simulink model "LKAS_AutoSave_DF_20220414_1924_SW62"  (R2018b)
settings: Solver=FixedStepDiscrete  StartTime=0.0  StopTime=10.0  FixedStep=0.01  RelTol=1e-3
model workspace (MAT data in the model file):
  MCOS : class17 (value not decoded)
  MCOS : class17 (value not decoded)
  MCOS : class17 (value not decoded)
  MCOS : class17 (value not decoded)
  MCOS : class17 (value not decoded)
  MCOS : class17 (value not decoded)
  MCOS : class17 (value not decoded)
  MCOS : class17 (value not decoded)
  MCOS : class17 (value not decoded)
  MCOS : class17 (value not decoded)
  MCOS : class17 (value not decoded)
  MCOS : class17 (value not decoded)
  MCOS : class17 (value not decoded)
  MCOS : class17 (value not decoded)
  MCOS : class17 (value not decoded)
  MCOS : class17 (value not decoded)
  MCOS : class17 (value not decoded)
  MCOS : class17 (value not decoded)
  MCOS : class17 (value not decoded)
  MCOS : class17 (value not decoded)
  MCOS : class17 (value not decoded)
  MCOS : class17 (value not decoded)
  MCOS : class17 (value not decoded)
  MCOS : class17 (value not decoded)
  MCOS : class17 (value not decoded)
  MCOS : class17 (value not decoded)
  MCOS : class17 (value not decoded)
  MCOS : class17 (value not decoded)
  MCOS : class17 (value not decoded)
  MCOS : class17 (value not decoded)
  MCOS : class17 (value not decoded)
  MCOS : class17 (value not decoded)
  MCOS : class17 (value not decoded)
  MCOS : class17 (value not decoded)
  MCOS : class17 (value not decoded)
  MCOS : class17 (value not decoded)
  MCOS : class17 (value not decoded)
  MCOS : class17 (value not decoded)
  MCOS : class17 (value not decoded)
  MCOS : class17 (value not decoded)
  MCOS : class17 (value not decoded)
  MCOS : class17 (value not decoded)
  MCOS : class17 (value not decoded)
  MCOS : class17 (value not decoded)
  MCOS : class17 (value not decoded)
  MCOS : class17 (value not decoded)
  MCOS : class17 (value not decoded)
  MCOS : class17 (value not decoded)
  MCOS : class17 (value not decoded)
  MCOS : class17 (value not decoded)
  MCOS : class17 (value not decoded)
  MCOS : class17 (value not decoded)
  MCOS : class17 (value not decoded)
  MCOS : class17 (value not decoded)
  MCOS : class17 (value not decoded)
  MCOS : class17 (value not decoded)
  MCOS : class17 (value not decoded)
  MCOS : class17 (value not decoded)
  MCOS : class17 (value not decoded)
  MCOS : class17 (value not decoded)
  MCOS : class17 (value not decoded)
  MCOS : class17 (value not decoded)
  MCOS : class17 (value not decoded)
  MCOS : class17 (value not decoded)
  MCOS : class17 (value not decoded)
  MCOS : class17 (value not decoded)
  MCOS : class17 (value not decoded)
  MCOS : class17 (value not decoded)
  MCOS : class17 (value not decoded)
  MCOS : class17 (value not decoded)
  MCOS : class17 (value not decoded)
  MCOS : class17 (value not decoded)
  MCOS : class17 (value not decoded)
  MCOS : class17 (value not decoded)
  MCOS : class17 (value not decoded)
  MCOS : class17 (value not decoded)
  MCOS : class17 (value not decoded)
  MCOS : class17 (value not decoded)
  MCOS : class17 (value not decoded)
  MCOS : class17 (value not decoded)
  MCOS : class17 (value not decoded)
  MCOS : class17 (value not decoded)
  MCOS : class17 (value not decoded)
  MCOS : class17 (value not decoded)
  MCOS : class17 (value not decoded)
  MCOS : class17 (value not decoded)
  MCOS : class17 (value not decoded)
  MCOS : class17 (value not decoded)
  MCOS : class17 (value not decoded)
  MCOS : class17 (value not decoded)
  MCOS : class17 (value not decoded)
  MCOS : class17 (value not decoded)
  MCOS : class17 (value not decoded)
  MCOS : class17 (value not decoded)
  MCOS : class17 (value not decoded)
  MCOS : class17 (value not decoded)
  MCOS : class17 (value not decoded)
  MCOS : class17 (value not decoded)
  MCOS : class17 (value not decoded)
  MCOS : class17 (value not decoded)
  MCOS : class17 (value not decoded)
  MCOS : class17 (value not decoded)
  MCOS : class17 (value not decoded)
  MCOS : class17 (value not decoded)
  MCOS : class17 (value not decoded)
  MCOS : class17 (value not decoded)
  MCOS : class17 (value not decoded)
  MCOS : class17 (value not decoded)
  MCOS : class17 (value not decoded)
undefined symbols (not defined in the file): LKA_CarWidth, LKA_SampleTime, LKA_StrRatio_C, LKA_Veh2CamL_C, LKA_Veh2CamW_C, LKA_WhlBaseL_C, LL_CompHdAg_C, LL_CompSWA_C, LL_CrvtPrvwT_C, LL_DesDvt_C, LL_DvtComp_C, LL_DvtPrvwT_C, LL_DvtSpdDet_vDvtSpdMin_C, LL_HandsOff_ExitTime, LL_HandsOff_TextTime, LL_HandsOff_WarnTime, LL_HdAgExT_C, LL_HdAgPrvwT_C, LL_LAccMax_C, LL_LAccRMax_C, LL_LDW_EarliestWarnLine_C, LL_LDW_LatestWarnLine_C, LL_LDWS_SUPPRESS_HEADING, LL_LFClb_TFC_FfCtlRatio_C, LL_LFClb_TFC_KdBalance_C, LL_LFClb_TFC_KdMaxSWA_C, LL_LFClb_TFC_KdV1_C, LL_LFClb_TFC_KdV2_C, LL_LFClb_TFC_KdVehSpdLwr_C, LL_LFClb_TFC_KdVehSpdUpr_C, LL_LFClb_TFC_Ki_C, LL_LFClb_TFC_KiMaxSWA_C, LL_LFClb_TFC_Kp_C, LL_LFClb_TFC_KpKlat_C, LL_LFClb_TFC_KpV1_C, LL_LFClb_TFC_KpV2_C, LL_LFClb_TFC_KpVehSpdLwr_C, LL_LFClb_TFC_KpVehSpdUpr_C, LL_LFClb_TFC_PrvwT_C, LL_LKA_EarliestWarnLine_C, LL_LKA_EnableLine_DvtMax, LL_LKA_EnableLine_DvtMin, LL_LKA_EnableLine_Max, LL_LKA_LatestWarnLine_C, LL_LKAExPrcs_ExitC0Dvt, LL_LKAExPrcs_ExitC0Swt, LL_LKAExPrcs_tiExitDelayTime3, LL_LKAExPrcs_tiExitTime1, LL_LKAExPrcs_tiExitTime2, LL_LKAExPrcs_tiExitTime3, LL_LKAS_OUT_OF_CONTROL_LAT_VEL, LL_LKAS_OUT_OF_CONTROL_TTLC, LL_LKASWASyn_M0, LL_LKASWASyn_M1, LL_LKASWASyn_M2, LL_LKASWASyn_M3D, LL_LKASWASyn_M3K_DT, LL_LKASWASyn_M3K_MSD, LL_LKASWASyn_M4K, LL_LKASWASyn_SWAaddMax ... (+50)
libraries: simulink x234, canmsglib x6, dspstat3 x3, simulink_extras x1
(part 12 of 17)

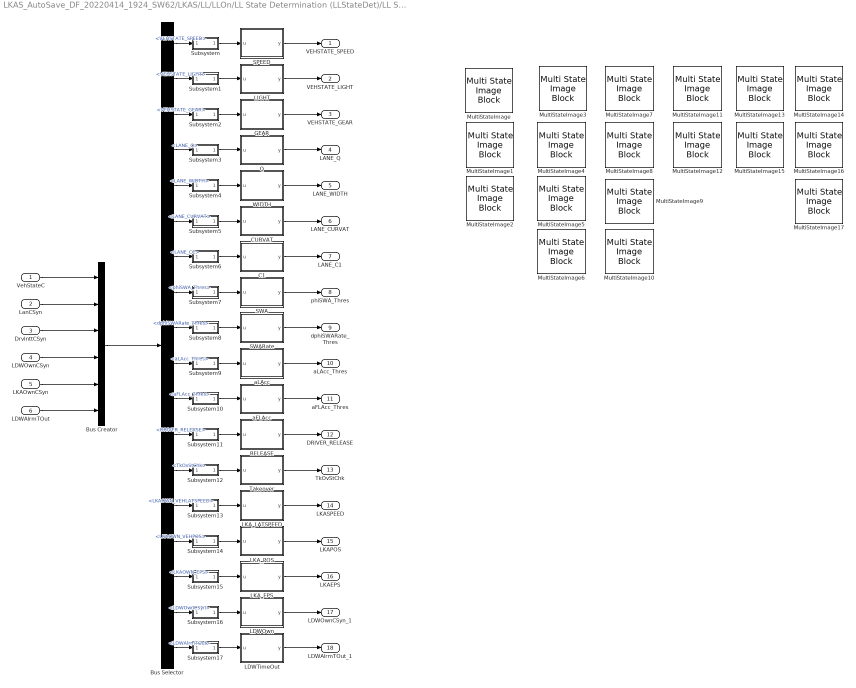
== system LKAS_AutoSave_DF_20220414_1924_SW62/LKAS/LL/LLOn/LL State Determination (LLStateDet)/LL State Machine Conditions (LLSMCon)/Disable Condition (DisblC)/Subsystem ==
  VehStateC : Inport
  LanCSyn : Inport  Port=2
  DrvInttCSyn : Inport  Port=3
  LDWOwnCSyn : Inport  Port=4
  LKAOwnCSyn : Inport  Port=5
  LDWAlrmTOut : Inport  Port=6
  Bus Creator : BusCreator  Inputs=6
  Bus Selector : BusSelector  OutputSignals=VehStateC.VEHSTATE_SPEED,VehStateC.VEHSTATE_LIGHT,VehStateC.VEHSTATE_GEAR,LaneCSyn.LANE_Q,LaneCSyn.LANE_WIDTH,LaneCSyn.LANE_CURVAT,LaneCSyn.LANE_C1,DrvInttCSyn.DrvActnDet.phiSWA_Thres,DrvInttCSyn.DrvActnDet.dphiSWARate_Thres,DrvInttCSyn.DrvActnDet.aLAcc_Thres,DrvInttCSyn.DrvActnDet.aFLAcc_Thres,DrvInttCSyn.DRIVER_RELEASE,DrvInttCSyn.TkOvStChk,LKAOwnSyn.LKAOWN_VEHLATSPEED,LKAOwnSyn.LKAOWN_VEHPOS,LKAOwnSyn.LKAOWN_EPS,LDWOwnCSyn,LDWAlrmTOut
  C1 : MATLAB Function  TreatAsAtomicUnit=on
  CURVAT : MATLAB Function  TreatAsAtomicUnit=on
  GEAR : MATLAB Function  TreatAsAtomicUnit=on
  LDWOwn : MATLAB Function  TreatAsAtomicUnit=on
  LDWTimeOut : MATLAB Function  TreatAsAtomicUnit=on
  LIGHT : MATLAB Function  TreatAsAtomicUnit=on
  LKA_EPS : MATLAB Function  TreatAsAtomicUnit=on
  LKA_LATSPEED : MATLAB Function  TreatAsAtomicUnit=on
  LKA_POS : MATLAB Function  TreatAsAtomicUnit=on
  MultiStateImage : MultiStateImageBlock  WebBlockId=3772
  MultiStateImage1 : MultiStateImageBlock  WebBlockId=3773
  MultiStateImage10 : MultiStateImageBlock  WebBlockId=3774
  MultiStateImage11 : MultiStateImageBlock  WebBlockId=3775
  MultiStateImage12 : MultiStateImageBlock  WebBlockId=3776
  MultiStateImage13 : MultiStateImageBlock  WebBlockId=3777
  MultiStateImage14 : MultiStateImageBlock  WebBlockId=3778
  MultiStateImage15 : MultiStateImageBlock  WebBlockId=3779
  MultiStateImage16 : MultiStateImageBlock  WebBlockId=3780
  MultiStateImage17 : MultiStateImageBlock  WebBlockId=3781
  MultiStateImage2 : MultiStateImageBlock  WebBlockId=3782
  MultiStateImage3 : MultiStateImageBlock  WebBlockId=3783
  MultiStateImage4 : MultiStateImageBlock  WebBlockId=3784
  MultiStateImage5 : MultiStateImageBlock  WebBlockId=3785
  MultiStateImage6 : MultiStateImageBlock  WebBlockId=3786
  MultiStateImage7 : MultiStateImageBlock  WebBlockId=3787
  MultiStateImage8 : MultiStateImageBlock  WebBlockId=3788
  MultiStateImage9 : MultiStateImageBlock  WebBlockId=3789
  Q : MATLAB Function  TreatAsAtomicUnit=on
  RELEASE : MATLAB Function  TreatAsAtomicUnit=on
  SPEED : MATLAB Function  TreatAsAtomicUnit=on
  SWA : MATLAB Function  TreatAsAtomicUnit=on
  SWARate : MATLAB Function  TreatAsAtomicUnit=on
  Subsystem : Subsystem
  Subsystem1 : Subsystem
  Subsystem10 : Subsystem
  Subsystem11 : Subsystem
  Subsystem12 : Subsystem
  Subsystem13 : Subsystem
  Subsystem14 : Subsystem
  Subsystem15 : Subsystem
  Subsystem16 : Subsystem
  Subsystem17 : Subsystem
  Subsystem2 : Subsystem
  Subsystem3 : Subsystem
  Subsystem4 : Subsystem
  Subsystem5 : Subsystem
  Subsystem6 : Subsystem
  Subsystem7 : Subsystem
  Subsystem8 : Subsystem
  Subsystem9 : Subsystem
  Takeover : MATLAB Function  TreatAsAtomicUnit=on
  WIDTH : MATLAB Function  TreatAsAtomicUnit=on
  aFLAcc : MATLAB Function  TreatAsAtomicUnit=on
  aLAcc : MATLAB Function  TreatAsAtomicUnit=on
  VEHSTATE_SPEED : Outport
  VEHSTATE_LIGHT : Outport  Port=2
  VEHSTATE_GEAR : Outport  Port=3
  LANE_Q : Outport  Port=4
  LANE_WIDTH : Outport  Port=5
  LANE_CURVAT : Outport  Port=6
  LANE_C1 : Outport  Port=7
  phiSWA_Thres : Outport  Port=8
  dphiSWARate_Thres : Outport  Port=9
  aLAcc_Thres : Outport  Port=10
  aFLAcc_Thres : Outport  Port=11
  DRIVER_RELEASE : Outport  Port=12
  TkOvStChk : Outport  Port=13
  LKASPEED : Outport  Port=14
  LKAPOS : Outport  Port=15
  LKAEPS : Outport  Port=16
  LDWOwnCSyn_1 : Outport  Port=17
  LDWAlrmTOut_1 : Outport  Port=18
  wires:
  Bus Selector/16 -> Subsystem15/1(in1)  "<LKAOWN_EPS>"
  Subsystem15/1(Out1) -> LKA_EPS/1(u)
  LKA_EPS/1(y) -> LKAEPS/1
  Bus Selector/14 -> Subsystem13/1(in1)  "<LKAOWN_VEHLATSPEED>"
  Subsystem13/1(Out1) -> LKA_LATSPEED/1(u)
  LKA_LATSPEED/1(y) -> LKASPEED/1
  Subsystem17/1(Out1) -> LDWTimeOut/1(u)
  Subsystem14/1(Out1) -> LKA_POS/1(u)
  Subsystem16/1(Out1) -> LDWOwn/1(u)
  Subsystem11/1(Out1) -> RELEASE/1(u)
  Subsystem12/1(Out1) -> Takeover/1(u)
  Subsystem10/1(Out1) -> aFLAcc/1(u)
  Subsystem9/1(Out1) -> aLAcc/1(u)
  Subsystem8/1(Out1) -> SWARate/1(u)
  Subsystem7/1(Out1) -> SWA/1(u)
  Subsystem6/1(Out1) -> C1/1(u)
  Subsystem5/1(Out1) -> CURVAT/1(u)
  Subsystem4/1(Out1) -> WIDTH/1(u)
  Subsystem3/1(Out1) -> Q/1(u)
  Subsystem2/1(Out1) -> GEAR/1(u)
  Subsystem1/1(Out1) -> LIGHT/1(u)
  Subsystem/1(Out1) -> SPEED/1(u)
  Bus Selector/1 -> Subsystem/1(in1)  "<VEHSTATE_SPEED>"
  SPEED/1(y) -> VEHSTATE_SPEED/1
  LIGHT/1(y) -> VEHSTATE_LIGHT/1
  GEAR/1(y) -> VEHSTATE_GEAR/1
  aLAcc/1(y) -> aLAcc_Thres/1
  WIDTH/1(y) -> LANE_WIDTH/1
  LDWTimeOut/1(y) -> LDWAlrmTOut_1/1
  SWA/1(y) -> phiSWA_Thres/1
  aFLAcc/1(y) -> aFLAcc_Thres/1
  LDWAlrmTOut/1 -> Bus Creator/6
  Bus Selector/6 -> Subsystem5/1(in1)  "<LANE_CURVAT>"
  RELEASE/1(y) -> DRIVER_RELEASE/1
  SWARate/1(y) -> dphiSWARate_Thres/1
  Bus Selector/3 -> Subsystem2/1(in1)  "<VEHSTATE_GEAR>"
  LDWOwnCSyn/1 -> Bus Creator/4
  DrvInttCSyn/1 -> Bus Creator/3
  Bus Selector/5 -> Subsystem4/1(in1)  "<LANE_WIDTH>"
  C1/1(y) -> LANE_C1/1
  LanCSyn/1 -> Bus Creator/2
  Takeover/1(y) -> TkOvStChk/1
  Bus Selector/7 -> Subsystem6/1(in1)  "<LANE_C1>"
  Bus Selector/9 -> Subsystem8/1(in1)  "<dphiSWARate_Thres>"
  Bus Selector/2 -> Subsystem1/1(in1)  "<VEHSTATE_LIGHT>"
  Q/1(y) -> LANE_Q/1
  CURVAT/1(y) -> LANE_CURVAT/1
  Bus Selector/12 -> Subsystem11/1(in1)  "<DRIVER_RELEASE>"
  Bus Selector/10 -> Subsystem9/1(in1)  "<aLAcc_Thres>"
  Bus Selector/11 -> Subsystem10/1(in1)  "<aFLAcc_Thres>"
  Bus Selector/15 -> Subsystem14/1(in1)  "<LKAOWN_VEHPOS>"
  LDWOwn/1(y) -> LDWOwnCSyn_1/1
  LKA_POS/1(y) -> LKAPOS/1
  Bus Selector/18 -> Subsystem17/1(in1)  "<LDWAlrmTOut>"
  Bus Selector/4 -> Subsystem3/1(in1)  "<LANE_Q>"
  VehStateC/1 -> Bus Creator/1
  Bus Creator/1 -> Bus Selector/1
  Bus Selector/17 -> Subsystem16/1(in1)  "<LDWOwnCSyn>"
  LKAOwnCSyn/1 -> Bus Creator/5
  Bus Selector/8 -> Subsystem7/1(in1)  "<phiSWA_Thres>"
  Bus Selector/13 -> Subsystem12/1(in1)  "<TkOvStChk>"

== system LKAS_AutoSave_DF_20220414_1924_SW62/LKAS/LL/LLOn/LL State Determination (LLStateDet)/LL State Machine Conditions (LLSMCon)/Disable Condition (DisblC)/Subsystem1 ==
  VehStateC : Inport
  LaneCSyn : Inport  Port=2
  DrvInttCSyn : Inport  Port=3
  LDWOwnCSyn : Inport  Port=4
  LKAOwnCSyn : Inport  Port=5
  LDWAlrmTOut : Inport  Port=6
  Bus Creator : BusCreator  Inputs=6
  Bus Selector : BusSelector  OutputSignals=VehStateC.VEHSTATE_SPEED,VehStateC.VEHSTATE_LIGHT,VehStateC.VEHSTATE_GEAR,LaneCSyn.LANE_Q,LaneCSyn.LANE_WIDTH,LaneCSyn.LANE_CURVAT,LaneCSyn.LANE_C1,DrvInttCSyn.DrvActnDet.phiSWA_Thres,DrvInttCSyn.DrvActnDet.dphiSWARate_Thres,DrvInttCSyn.DrvActnDet.aLAcc_Thres,DrvInttCSyn.DrvActnDet.aFLAcc_Thres,DrvInttCSyn.DRIVER_RELEASE,DrvInttCSyn.TkOvStChk,LKAOwnCSyn.LKAOWN_VEHLATSPEED,LKAOwnCSyn.LKAOWN_VEHPOS,LKAOwnCSyn.LKAOWN_EPS,LDWOwnCSyn,LDWAlrmTOutSyn
  Disable Reason : MATLAB Function  TreatAsAtomicUnit=on
  Mux : Mux  Inputs=18
  DisableReason : Outport
  wires:
  Disable Reason/1(y) -> DisableReason/1  "Disable_Reason"
  Mux/1 -> Disable Reason/1(u)
  Bus Selector/16 -> Mux/16  "<LKAOWN_EPS>"
  Bus Selector/14 -> Mux/14  "<LKAOWN_VEHLATSPEED>"
  Bus Selector/1 -> Mux/1  "<VEHSTATE_SPEED>"
  LDWAlrmTOut/1 -> Bus Creator/6
  Bus Selector/6 -> Mux/6  "<LANE_CURVAT>"
  Bus Selector/3 -> Mux/3  "<VEHSTATE_GEAR>"
  LDWOwnCSyn/1 -> Bus Creator/4
  DrvInttCSyn/1 -> Bus Creator/3
  Bus Selector/5 -> Mux/5  "<LANE_WIDTH>"
  LaneCSyn/1 -> Bus Creator/2
  Bus Selector/7 -> Mux/7  "<LANE_C1>"
  Bus Selector/9 -> Mux/9  "<dphiSWARate_Thres>"
  Bus Selector/2 -> Mux/2  "<VEHSTATE_LIGHT>"
  Bus Selector/12 -> Mux/12  "<DRIVER_RELEASE>"
  Bus Selector/10 -> Mux/10  "<aLAcc_Thres>"
  Bus Selector/11 -> Mux/11  "<aFLAcc_Thres>"
  Bus Selector/15 -> Mux/15  "<LKAOWN_VEHPOS>"
  Bus Selector/18 -> Mux/18  "<LDWAlrmTOutSyn>"
  Bus Selector/4 -> Mux/4  "<LANE_Q>"
  VehStateC/1 -> Bus Creator/1
  Bus Creator/1 -> Bus Selector/1
  Bus Selector/17 -> Mux/17  "<LDWOwnCSyn>"
  LKAOwnCSyn/1 -> Bus Creator/5
  Bus Selector/8 -> Mux/8  "<phiSWA_Thres>"
  Bus Selector/13 -> Mux/13  "<TkOvStChk>"

== system LKAS_AutoSave_DF_20220414_1924_SW62/LKAS/LL/LLOn/LL State Determination (LLStateDet)/LL State Machine Conditions (LLSMCon)/Disable Condition (DisblC)/Vehicle State Condition (VehStateC) ==
  LKA_Mode : Inport
  InInfoSyn : Inport  Port=2
  LLClb : Inport  Port=3
  LLState : Inport  Port=4
  Accelerate Validity Disable Condition (AccValidDC) : Subsystem  Description=|
      | Block Name: Emergency Light Enable Condition
      | Ab.: EmgcyLghtEC
      | No.: 1.1.1.2.1.3
      | Rev: 0.0.1
      | Update Date: 19-3-26
  Bus Creator : BusCreator  Inputs=3
  Bus Selector : BusSelector  OutputSignals=bsVehMovInfo.ESC_VehSpd,bsVehMovInfo.ESC_LatAcc_Valid,bsVehMovInfo.ESC_LonAcc_Valid,bsBCMInfo,bsPTState.TCU_ActualGear
  Bus Selector1 : BusSelector  OutputSignals=bsLLSMConClb.DisblCClb.LL_MAX_LDWS_SPEED_DISABLE,bsLLSMConClb.DisblCClb.LL_MAX_LKAS_SPEED_DISABLE,bsLLSMConClb.DisblCClb.LL_MIN_LKAS_SPEED_DISABLE,bsLLSMConClb.DisblCClb.LL_SingleLane_Disable_Swt
  Bus Selector2 : BusSelector  OutputSignals=LKA_State
  Emergency Light Enable Condition (EmgcyLghtEC) : Subsystem  Description=|
      | Block Name: Emergency Light Enable Condition
      | Ab.: EmgcyLghtEC
      | No.: 1.1.1.2.1.3
      | Rev: 0.0.1
      | Update Date: 19-3-26
  Gear Disable Condition (GearDC) : Subsystem  Description=|
      | Block Name: Gear Disable Condition
      | Ab.: GearDC
      | No.: 1.1.1.3.1.4
      | Rev: 0.0.1
      | Update Date: 19-3-26
  Vehicle Speed Disable Condition (VehSpdDC) : Subsystem  Description=|
      | Block Name: Vehicle Speed Disable Condition
      | Ab.: VehSpdDC
      | No.: 1.1.1.3.1.1
      | Rev: 0.0.1
      | Update Date: 19-3-26
  Vehicle State Condition Synthesis (VehStateCSyn) : Subsystem  Description=|
      | Block Name: Vehicle State Condition Synthesis
      | Ab.: VehStateCSyn
      | No.: 1.1.1.3.1.5
      | Rev: 0.0.1
      | Update Date: 19-3-26
  stVehStateC : Outport
  VehStateC : Outport  Port=2
  wires:
  Accelerate Validity Disable Condition (AccValidDC)/1(AccValidDC_stAccValidDCFlg) -> Vehicle State Condition Synthesis (VehStateCSyn)/2(AccValidDC_stAccValidDCFlg)  "ACC_VALID"
  Bus Selector/3 -> Accelerate Validity Disable Condition (AccValidDC)/2(ESC_LonAcc_Valid)  "<ESC_LonAcc_Valid>"
  Bus Selector/2 -> Accelerate Validity Disable Condition (AccValidDC)/1(ESC_LatAcc_Valid)  "<ESC_LatAcc_Valid>"
  LLState/1 -> Bus Selector2/1
  Bus Selector2/1 -> Emergency Light Enable Condition (EmgcyLghtEC)/3(EmgcyLghtEC_bsLLState)  "<LKA_State>"
  Bus Selector1/4 -> Emergency Light Enable Condition (EmgcyLghtEC)/2(EmgcyLghtEC_SingleLane_Disable_Swt)  "<LL_SingleLane_Disable_Swt>"
  Bus Creator/1 -> VehStateC/1  "VehStateC"
  Bus Selector/4 -> Emergency Light Enable Condition (EmgcyLghtEC)/1(EmgcyLghtEC_bsStLampState)  "<bsBCMInfo>"
  Gear Disable Condition (GearDC)/1(GearDC_stGearDCFlg) -> Bus Creator/3, Vehicle State Condition Synthesis (VehStateCSyn)/4(VehStateCSyn_stGearDCFlg)  "VEHSTATE_GEAR"
  Bus Selector/5 -> Gear Disable Condition (GearDC)/1(GearDC_TCU_ActualGear)  "<TCU_ActualGear>"
  Emergency Light Enable Condition (EmgcyLghtEC)/1(EmgcyLghtEC_stEmgcyLghtECFlg) -> Vehicle State Condition Synthesis (VehStateCSyn)/3(VehStateCSyn_stEmgcyLghtDCFlg), Bus Creator/2  "VEHSTATE_LIGHT"
  Bus Selector1/2 -> Vehicle Speed Disable Condition (VehSpdDC)/4(VehSpdDC_vLKAVehSpdMax_C)  "<LL_MAX_LKAS_SPEED_DISABLE>"
  Bus Selector1/3 -> Vehicle Speed Disable Condition (VehSpdDC)/5(VehSpdDC_vVehSpdMin_C)  "<LL_MIN_LKAS_SPEED_DISABLE>"
  LLClb/1 -> Bus Selector1/1
  LKA_Mode/1 -> Vehicle Speed Disable Condition (VehSpdDC)/1(VehSpdDC_stDACMode)
  Bus Selector1/1 -> Vehicle Speed Disable Condition (VehSpdDC)/3(VehSpdDC_vLDWVehSpdMax_C)  "<LL_MAX_LDWS_SPEED_DISABLE>"
  Vehicle Speed Disable Condition (VehSpdDC)/1(VehSpdDC_stVehSpdDCFlg) -> Vehicle State Condition Synthesis (VehStateCSyn)/1(VehStateCSyn_stVehSpdDCFlg), Bus Creator/1  "VEHSTATE_SPEED"
  Bus Selector/1 -> Vehicle Speed Disable Condition (VehSpdDC)/2(VehSpdDC_vVehSpd)  "<ESC_VehSpd>"
  Vehicle State Condition Synthesis (VehStateCSyn)/1(VehStateCSyn_stVehStateCSyn) -> stVehStateC/1  "VEHSTATE"
  InInfoSyn/1 -> Bus Selector/1

== system LKAS_AutoSave_DF_20220414_1924_SW62/LKAS/LL/LLOn/LL State Determination (LLStateDet)/LL State Machine Conditions (LLSMCon)/Enable Condition (EnaC)/Driver Intent Condition (DrvInttC) ==
  InInfoSyn : Inport
  LLClb : Inport  Port=2
  Abs{1..4} (4 alike) : Abs  OutDataTypeStr=single
  Bus Selector : BusSelector  OutputSignals=bsSWAInfo.SW_Angle,bsSWAInfo.SW_Angle_Speed,bsEPSInfo.EPS_SW_Trq,bsVehMovInfo.ESC_LatAcc,bsVehMovInfo.ESC_LonAcc
  Bus Selector1 : BusSelector  OutputSignals=bsLLSMConClb.EnaCClb.LL_MAX_STEER_ANGLE_ENABLE,bsLLSMConClb.EnaCClb.LL_MAX_STEER_SPEED_ENABLE,bsLLSMConClb.EnaCClb.LL_MAX_DRIVER_TORQUE_ENABLE,bsLLSMConClb.EnaCClb.LL_MAX_LAT_ACC_ENABLE,bsLLSMConClb.EnaCClb.LL_MAX_LONG_ACC_ENABLE,bsLLSMConClb.EnaCClb.LL_MAX_LONG_DECEL_ENABLE
  Interval Test Dynamic : simulink/Logic and Bit Operations/Interval Test Dynamic  IntervalClosedRight=off  IntervalClosedLeft=off  OutDataTypeStr=boolean
      settings: SourceProductName=Simulink  SourceProductBaseCode=SL
  Logical Operator3 : Logic  Inputs=5  AllPortsSameDT=off  OutDataTypeStr=boolean
  Relational Operator{,1..3} (4 alike) : RelationalOperator  Operator=<  OutDataTypeStr=boolean  RndMeth=Nearest
  Unary Minus : UnaryMinus
  stDrvInttC : Outport
  wires:
  Bus Selector/2 -> Abs3/1  "<SW_Angle_Speed>"
  Relational Operator/1 -> Logical Operator3/3
  Relational Operator1/1 -> Logical Operator3/1
  Abs2/1 -> Relational Operator1/1
  Abs3/1 -> Relational Operator2/1
  Relational Operator2/1 -> Logical Operator3/2
  Abs4/1 -> Relational Operator3/1
  Abs1/1 -> Relational Operator/1
  Unary Minus/1 -> Interval Test Dynamic/3
  Relational Operator3/1 -> Logical Operator3/4
  Interval Test Dynamic/1 -> Logical Operator3/5
  Logical Operator3/1 -> stDrvInttC/1  "DRIVERINT_ACTION"
  LLClb/1 -> Bus Selector1/1
  Bus Selector1/6 -> Unary Minus/1  "<LL_MAX_LONG_DECEL_ENABLE>"
  Bus Selector1/5 -> Interval Test Dynamic/1  "<LL_MAX_LONG_ACC_ENABLE>"
  Bus Selector1/4 -> Relational Operator3/2  "<LL_MAX_LAT_ACC_ENABLE>"
  Bus Selector1/3 -> Relational Operator/2  "<LL_MAX_DRIVER_TORQUE_ENABLE>"
  Bus Selector1/2 -> Relational Operator2/2  "<LL_MAX_STEER_SPEED_ENABLE>"
  Bus Selector1/1 -> Relational Operator1/2  "<LL_MAX_STEER_ANGLE_ENABLE>"
  Bus Selector/5 -> Interval Test Dynamic/2  "<ESC_LonAcc>"
  Bus Selector/4 -> Abs4/1  "<ESC_LatAcc>"
  Bus Selector/1 -> Abs2/1  "<SW_Angle>"
  Bus Selector/3 -> Abs1/1  "<EPS_SW_Trq>"
  InInfoSyn/1 -> Bus Selector/1

== system LKAS_AutoSave_DF_20220414_1924_SW62/LKAS/LL/LLOn/LL State Determination (LLStateDet)/LL State Machine Conditions (LLSMCon)/Enable Condition (EnaC)/Enable Condition Synthesis (EnaCSyn) ==
  LKA_Mode : Inport
  stVehStateC : Inport  Port=2
  stLaneC : Inport  Port=3
  stDrvInttC : Inport  Port=4
  stLDWOwnC : Inport  Port=5
  stLKAOwnC : Inport  Port=6
  Cast To Single : DataTypeConversion  OutDataTypeStr=uint8
  Cast To Single2 : DataTypeConversion  OutDataTypeStr=uint8
  If : If  NumInputs=2  IfExpression=(u1 ==1|u1==2)& u2 ==1
  If Action Subsystem : Subsystem  TreatAsAtomicUnit=on
  If Action Subsystem2 : Subsystem  TreatAsAtomicUnit=on
  If Action Subsystem3 : Subsystem  TreatAsAtomicUnit=on
  If Action Subsystem4 : Subsystem  TreatAsAtomicUnit=on
  If1 : If  NumInputs=2  IfExpression=u1 == 2 & u2
  Logical Operator1 : Logic  AllPortsSameDT=off  OutDataTypeStr=boolean
  Logical Operator2 : Logic  Inputs=3  AllPortsSameDT=off  OutDataTypeStr=boolean
  Logical Operator3 : Logic  AllPortsSameDT=off  OutDataTypeStr=boolean
  Merge : Merge
  Merge1 : Merge
  stLDWEnaCSyn : Outport
  stLKAEnaCSyn : Outport  Port=2
  wires:
  Cast To Single2/1 -> If1/2
  Cast To Single/1 -> If/2
  Logical Operator3/1 -> Cast To Single/1
  LKA_Mode/1 -> If/1, If1/1
  Logical Operator1/1 -> Cast To Single2/1
  If Action Subsystem4/1(Out) -> Merge1/2
  Merge1/1 -> stLKAEnaCSyn/1
  If1/2 -> If Action Subsystem4/Action
  If1/1 -> If Action Subsystem2/Action
  If Action Subsystem2/1(Out) -> Merge1/1
  If Action Subsystem3/1(Out) -> Merge/2
  stLKAOwnC/1 -> Logical Operator1/2
  Logical Operator2/1 -> Logical Operator3/2, Logical Operator1/1
  Merge/1 -> stLDWEnaCSyn/1
  stLDWOwnC/1 -> Logical Operator3/1
  If/2 -> If Action Subsystem3/Action
  If/1 -> If Action Subsystem/Action
  If Action Subsystem/1(Out) -> Merge/1
  stDrvInttC/1 -> Logical Operator2/3
  stLaneC/1 -> Logical Operator2/2
  stVehStateC/1 -> Logical Operator2/1

== system LKAS_AutoSave_DF_20220414_1924_SW62/LKAS/LL/LLOn/LL State Determination (LLStateDet)/LL State Machine Conditions (LLSMCon)/Enable Condition (EnaC)/LDW Own Condition (LDWOwnC) ==
  LKA_Mode : Inport
  LKAInPInfo : Inport  Port=2
  LLClb : Inport  Port=3
  Bus Selector : BusSelector  OutputSignals=LaneWidth,bsDvtInfo
  Bus Selector1 : BusSelector  OutputSignals=bsLLSMConClb.ActvCClb.LL_ThresDet_lDvtThresUprLDW,bsConstantClb.LKA_CarWidth
  LDW Own Condition Synthesis (LDWOwnCSyn) : Subsystem  Description=|
      | Block Name: LDW Own Condition Synthesis
      | Ab.: LDWOwnCSyn
      | No.: 1.1.1.2.4.2
      | Rev: 0.0.1
      | Update Date: 19-3-26
  Vehicle Position Check (VehPosChk) : Subsystem  Description=|
      | Block Name: Vehicle Position Check
      | Ab.: VehPosChk
      | No.: 1.1.1.2.4.1
      | Rev: 0.0.1
      | Update Date: 19-3-26
  stLDWOwnC : Outport
  wires:
  LKAInPInfo/1 -> Bus Selector/1
  Bus Selector1/2 -> Vehicle Position Check (VehPosChk)/4(VehPosChk_CarWidth)  "<LKA_CarWidth>"
  Bus Selector/1 -> Vehicle Position Check (VehPosChk)/1(VehPosChk_LaneWidth)  "<LaneWidth>"
  Bus Selector/2 -> Vehicle Position Check (VehPosChk)/2(VehPosChk_bsDvtInfo)  "<bsDvtInfo>"
  Bus Selector1/1 -> Vehicle Position Check (VehPosChk)/3(VehPosChk_lWarnLine_C)  "<LL_ThresDet_lDvtThresUprLDW>"
  LLClb/1 -> Bus Selector1/1
  LKA_Mode/1 -> LDW Own Condition Synthesis (LDWOwnCSyn)/1(LDWOwnCSyn_stDACMode)
  Vehicle Position Check (VehPosChk)/1(VehPosChk_stVehPosChk) -> LDW Own Condition Synthesis (LDWOwnCSyn)/2(LDWOwnCSyn_stVehPosChk)
  LDW Own Condition Synthesis (LDWOwnCSyn)/1(stLDWOwnC) -> stLDWOwnC/1  "stLDWOwnC"

== system LKAS_AutoSave_DF_20220414_1924_SW62/LKAS/LL/LLOn/LL State Determination (LLStateDet)/LL State Machine Conditions (LLSMCon)/Enable Condition (EnaC)/LKA Own Condition (LKAOwnC) ==
  LKA_Mode : Inport
  InInfoSyn : Inport  Port=2
  LKAInPInfo : Inport  Port=3
  LLClb : Inport  Port=4
  Bus Selector : BusSelector  OutputSignals=bsEPSInfo
  Bus Selector1 : BusSelector  OutputSignals=bsLLSMConClb.EnaCClb.LL_LKAS_OUT_OF_CONTROL_LAT_VEL,bsConstantClb.LKA_CarWidth,bsLLSMConClb.EnaCClb.LL_LKA_LatestWarnLine_C,bsLLSMConClb.EnaCClb.LL_LKA_EnableLine_Max,bsLLSMConClb.EnaCClb.LL_LKA_EnableLine_DvtMin,bsLLSMConClb.EnaCClb.LL_LKA_EnableLine_DvtMax,bsLLSMConClb.EnaCClb.LL_LKAS_OUT_OF_CONTROL_TTLC
  Bus Selector2 : BusSelector  OutputSignals=bsTTLCInfo,LaneWidth,bsDvtInfo
  EPS State Condition (EPSStC) : Subsystem  Description=|
      | Block Name: EPS State Condition
      | Ab.: EPSStC
      | No.: 1.1.1.2.5.1
      | Rev: 0.0.1
      | Update Date: 19-3-26
  Exit Lane Delay (ExLaneDel) : Subsystem  Description=|  Commented=on
      | Block Name: Exit Lane Delay
      | Ab.: ExLaneDel
      | No.: 1.1.1.2.5.5
      | Rev: 0.0.1
      | Update Date: 19-3-26
  LKA Own Condition Synthesis (LKAOwnCSyn) : Subsystem  Description=|
      | Block Name: LKA Own Condition Synthesis
      | Ab.: LKAOwnCSyn
      | No.: 1.1.1.2.5.6
      | Rev: 0.0.1
      | Update Date: 19-3-26
  Vehicle Lateral Speed Condition (VehLSpdC) : Subsystem  Description=|
      | Block Name: Vehicle Lateral Speed Condition
      | Ab.: VehLSpdC
      | No.: 1.1.1.2.5.3
      | Rev: 0.0.1
      | Update Date: 19-3-26
  Vehicle Position Check (VehPosChk)1 : Subsystem  Description=|
      | Block Name: Vehicle Position Check
      | Ab.: VehPosChk
      | No.: 1.1.1.2.4.1
      | Rev: 0.0.1
      | Update Date: 19-3-26
  stLKAOwnC : Outport
  wires:
  Bus Selector2/3 -> Vehicle Position Check (VehPosChk)1/2(VehPosChk_bsDvtInfo)  "<bsDvtInfo>"
  LKAInPInfo/1 -> Bus Selector2/1
  Bus Selector1/2 -> Vehicle Position Check (VehPosChk)1/3(VehPosChk_CarWidth)  "<LKA_CarWidth>"
  Bus Selector2/2 -> Vehicle Position Check (VehPosChk)1/1(VehPosChk_LaneWidth)  "<LaneWidth>"
  Bus Selector1/1 -> Vehicle Lateral Speed Condition (VehLSpdC)/2(VehLSpdC_vVehLSpdMax_C)  "<LL_LKAS_OUT_OF_CONTROL_LAT_VEL>"
  Bus Selector1/3 -> Vehicle Position Check (VehPosChk)1/4(VehPosChk_lWarnLineMin_C)  "<LL_LKA_LatestWarnLine_C>"
  Bus Selector1/7 -> Exit Lane Delay (ExLaneDel)/2(ExLaneDel_tiExLaneDelT)  "<LL_LKAS_OUT_OF_CONTROL_TTLC>"
  LLClb/1 -> Bus Selector1/1
  Vehicle Lateral Speed Condition (VehLSpdC)/1(VehLSpdC_stVehLSpdC) -> LKA Own Condition Synthesis (LKAOwnCSyn)/3(LKAOwnCSyn_stVehLSpdC)  "LKAOWN_VEHLSPD"
  Vehicle Position Check (VehPosChk)1/2(VehPosChk_stVehExLane) -> Exit Lane Delay (ExLaneDel)/1(ExLaneDel_stVehExLane)
  Exit Lane Delay (ExLaneDel)/1(ExLaneDel_stExLaneDel) -> LKA Own Condition Synthesis (LKAOwnCSyn)/5(LKAOwnCSyn_stExLaneDel)  "LKAOWN_EXITLANE"
  LKA_Mode/1 -> LKA Own Condition Synthesis (LKAOwnCSyn)/1(LKAOwnCSyn_stDACMode)
  EPS State Condition (EPSStC)/1(EPSStC_tfEPSCtlEC) -> LKA Own Condition Synthesis (LKAOwnCSyn)/2(LKAOwnCSyn_stEPSCtlEC)  "LKAOWN_EPS"
  Bus Selector/1 -> EPS State Condition (EPSStC)/1(EPSStC_bsEPSInfo)  "<bsEPSInfo>"
  Vehicle Position Check (VehPosChk)1/1(VehPosChk_stVehPosChk) -> LKA Own Condition Synthesis (LKAOwnCSyn)/4(LKAOwnCSyn_stVehPosChk)  "LKAOWN_VEHPOS"
  InInfoSyn/1 -> Bus Selector/1
  LKA Own Condition Synthesis (LKAOwnCSyn)/1(LKAOwnCSyn_stLKAPptyCSyn) -> stLKAOwnC/1  "LKAOWN"
  Bus Selector2/1 -> Vehicle Lateral Speed Condition (VehLSpdC)/1(VehLSpdC_bsTTLCInfo)  "<bsTTLCInfo>"
  Bus Selector1/4 -> Vehicle Position Check (VehPosChk)1/5(VehPosChk_LKAline_Enable_Max)  "<LL_LKA_EnableLine_Max>"
  Bus Selector1/5 -> Vehicle Position Check (VehPosChk)1/6(VehPosChk_LKAline_Enable_DvtMin)  "<LL_LKA_EnableLine_DvtMin>"
  Bus Selector1/6 -> Vehicle Position Check (VehPosChk)1/7(VehPosChk_LKAline_Enable_DvtMax)  "<LL_LKA_EnableLine_DvtMax>"

== system LKAS_AutoSave_DF_20220414_1924_SW62/LKAS/LL/LLOn/LL State Determination (LLStateDet)/LL State Machine Conditions (LLSMCon)/Enable Condition (EnaC)/Lane Condition (LaneC) ==
  InInfoSyn : Inport
  LKAInPInfo : Inport  Port=2
  LLClb : Inport  Port=3
  Bus Selector : BusSelector  OutputSignals=bsLaneInfo.bsL0Info.L0_Q,bsLaneInfo.bsR0Info.R0_Q,bsLaneInfo.bsL0Info.L0_C1,bsLaneInfo.bsR0Info.R0_C1
  Bus Selector1 : BusSelector  OutputSignals=bsLLSMConClb.EnaCClb.LL_MAX_LANE_WIDTH_ENABLE,bsLLSMConClb.EnaCClb.LL_MIN_LANE_WIDTH_ENABLE,bsLLSMConClb.EnaCClb.LL_MAX_SYSTEM_CURVATURE_ENABLE
  Bus Selector2 : BusSelector  OutputSignals=LaneWidth,bsPrCrvtInfo.crPrvwCrvt
  Lane C1 Detection (LaneC1Det) : Subsystem  Description=|
      | Block Name: Lane Width Detection
      | Ab.: LaneWDet
      | No.: 1.1.1.3.2.2
      | Rev: 0.0.1
      | Update Date: 19-3-26
  Lane Condition Synthesis (LaneCSyn) : Subsystem  Description=|
      | Block Name: Lane Condition Synthesis
      | Ab.: LaneCSyn
      | No.: 1.1.1.2.2.4
      | Rev: 0.0.1
      | Update Date: 19-3-26
  Lane Curvature Detection (LaneCrvtDet) : Subsystem  Description=|
      | Block Name: Lane Curvature Detection
      | Ab.: LaneCrvtDet
      | No.: 1.1.1.2.2.3
      | Rev: 0.0.1
      | Update Date: 19-3-26
  Lane Quality Enable Condition (LaneQlEC) : Subsystem  Description=|
      | Block Name: Lane Quality Enable Condition
      | Ab.: LaneQlEC
      | No.: 1.1.1.2.2.1
      | Rev: 0.0.1
      | Update Date: 19-3-26
  Lane Width Detection (LaneWDet) : Subsystem  Description=|
      | Block Name: Lane Width Detection
      | Ab.: LaneWDet
      | No.: 1.1.1.2.2.2
      | Rev: 0.0.1
      | Update Date: 19-3-26
  stLaneC : Outport
  wires:
  LKAInPInfo/1 -> Bus Selector2/1
  Lane C1 Detection (LaneC1Det)/1(stLaneC1DetFlg) -> Lane Condition Synthesis (LaneCSyn)/4(stLaneC1DetFlg)  "stLaneC1DetFlg"
  Bus Selector/4 -> Lane C1 Detection (LaneC1Det)/2(R0_C1)  "<R0_C1>"
  Bus Selector/3 -> Lane C1 Detection (LaneC1Det)/1(L0_C1)  "<L0_C1>"
  Bus Selector2/1 -> Lane Width Detection (LaneWDet)/1(LaneWidth)  "<LaneWidth>"
  Lane Condition Synthesis (LaneCSyn)/1(stLaneC_LKA) -> stLaneC/1
  Bus Selector2/2 -> Lane Curvature Detection (LaneCrvtDet)/1(crPrvwCrvt)  "<crPrvwCrvt>"
  Bus Selector1/2 -> Lane Width Detection (LaneWDet)/3(LL_MIN_LANE_WIDTH_ENABLE)  "<LL_MIN_LANE_WIDTH_ENABLE>"
  LLClb/1 -> Bus Selector1/1
  Bus Selector1/3 -> Lane Curvature Detection (LaneCrvtDet)/2(LL_MAX_SYSTEM_CURVATURE_ENABLE)  "<LL_MAX_SYSTEM_CURVATURE_ENABLE>"
  Bus Selector1/1 -> Lane Width Detection (LaneWDet)/2(LL_MAX_LANE_WIDTH_ENABLE)  "<LL_MAX_LANE_WIDTH_ENABLE>"
  Lane Curvature Detection (LaneCrvtDet)/1(stLaneCrvtDetFlg) -> Lane Condition Synthesis (LaneCSyn)/3(stLaneCrvtDetFlg)  "stLaneCrvtDetFlg"
  Lane Width Detection (LaneWDet)/1(stLaneWDetFlg) -> Lane Condition Synthesis (LaneCSyn)/2(stLaneWDetFlg)  "stLaneWDetFlg"
  Lane Quality Enable Condition (LaneQlEC)/1(stLaneQlECFlg) -> Lane Condition Synthesis (LaneCSyn)/1(stLaneQlECFlg)  "stLaneQlECFlg"
  Bus Selector/2 -> Lane Quality Enable Condition (LaneQlEC)/2(R0_Q)  "<R0_Q>"
  Bus Selector/1 -> Lane Quality Enable Condition (LaneQlEC)/1(L0_Q)  "<L0_Q>"
  InInfoSyn/1 -> Bus Selector/1

== system LKAS_AutoSave_DF_20220414_1924_SW62/LKAS/LL/LLOn/LL State Determination (LLStateDet)/LL State Machine Conditions (LLSMCon)/Enable Condition (EnaC)/Vehicle State Condition (VehStateC) ==
  LKA_Mode : Inport
  InInfoSyn : Inport  Port=2
  LLClb : Inport  Port=3
  Accelerate Validity Enable Condition (AccValidEC) : Subsystem  Description=|
      | Block Name: Emergency Light Enable Condition
      | Ab.: EmgcyLghtEC
      | No.: 1.1.1.2.1.3
      | Rev: 0.0.1
      | Update Date: 19-3-26
  Bus Selector : BusSelector  OutputSignals=bsVehMovInfo.ESC_VehSpd,bsVehMovInfo.ESC_LatAcc_Valid,bsVehMovInfo.ESC_LonAcc_Valid,bsBCMInfo,bsPTState
  Bus Selector1 : BusSelector  OutputSignals=bsLLSMConClb.EnaCClb.LL_MAX_LDWS_SPEED_ENABLE,bsLLSMConClb.EnaCClb.LL_MAX_LKAS_SPEED_ENABLE,bsLLSMConClb.EnaCClb.LL_MIN_LKAS_SPEED_ENABLE
  Emergency Light Enable Condition (EmgcyLghtEC) : Subsystem  Description=|
      | Block Name: Emergency Light Enable Condition
      | Ab.: EmgcyLghtEC
      | No.: 1.1.1.2.1.3
      | Rev: 0.0.1
      | Update Date: 19-3-26
  Gear Enable Condition (GearEC) : Subsystem  Description=|
      | Block Name: Gear Enable Condition
      | Ab.: GearEC
      | No.: 1.1.1.2.1.4
      | Rev: 0.0.1
      | Update Date: 19-3-26
  Vehicle Speed Enable Condition (VehSpdEC) : Subsystem  Description=|
      | Block Name: Vehicle Speed Enable Condition
      | Ab.: VehSpdEC
      | No.: 1.1.1.2.1.1
      | Rev: 0.0.1
      | Update Date: 19-3-26
  Vehicle State Condition Synthesis (VehStateCSyn) : Subsystem  Description=|
      | Block Name: Vehicle State Condition Synthesis
      | Ab.: VehStateCSyn
      | No.: 1.1.1.2.1.5
      | Rev: 0.0.1
      | Update Date: 19-3-26
  stVehStateC : Outport
  wires:
  Bus Selector/3 -> Accelerate Validity Enable Condition (AccValidEC)/2(ESC_LonAcc_Valid)  "<ESC_LonAcc_Valid>"
  Bus Selector/2 -> Accelerate Validity Enable Condition (AccValidEC)/1(ESC_LatAcc_Valid)  "<ESC_LatAcc_Valid>"
  Accelerate Validity Enable Condition (AccValidEC)/1(AccValidDC_stAccValidECFlg) -> Vehicle State Condition Synthesis (VehStateCSyn)/2(AccValidDC_stAccValidECFlg)  "ACC_VALID"
  Emergency Light Enable Condition (EmgcyLghtEC)/1(stEmgcyLghtECFlg) -> Vehicle State Condition Synthesis (VehStateCSyn)/3(stEmgcyLghtECFlg)  "stEmgcyLghtECFlg"
  Bus Selector/4 -> Emergency Light Enable Condition (EmgcyLghtEC)/1(bsBCMInfo)  "<bsBCMInfo>"
  Bus Selector/5 -> Gear Enable Condition (GearEC)/1(bsPTState)  "<bsPTState>"
  LKA_Mode/1 -> Vehicle Speed Enable Condition (VehSpdEC)/1(LKA_Mode)
  LLClb/1 -> Bus Selector1/1
  Bus Selector1/2 -> Vehicle Speed Enable Condition (VehSpdEC)/4(LL_MAX_LKAS_SPEED_ENABLE)  "<LL_MAX_LKAS_SPEED_ENABLE>"
  Bus Selector1/3 -> Vehicle Speed Enable Condition (VehSpdEC)/5(LL_MIN_LKAS_SPEED_ENABLE)  "<LL_MIN_LKAS_SPEED_ENABLE>"
  Bus Selector1/1 -> Vehicle Speed Enable Condition (VehSpdEC)/3(LL_MAX_LDWS_SPEED_ENABLE)  "<LL_MAX_LDWS_SPEED_ENABLE>"
  Bus Selector/1 -> Vehicle Speed Enable Condition (VehSpdEC)/2(ESC_VehSpd)  "<ESC_VehSpd>"
  Vehicle State Condition Synthesis (VehStateCSyn)/1(stVehStateC) -> stVehStateC/1  "stVehStateC"
  Gear Enable Condition (GearEC)/1(stGearECFlg) -> Vehicle State Condition Synthesis (VehStateCSyn)/4(stGearECFlg)  "stGearECFlg"
  InInfoSyn/1 -> Bus Selector/1
  Vehicle Speed Enable Condition (VehSpdEC)/1(stVehSpdECFlg) -> Vehicle State Condition Synthesis (VehStateCSyn)/1(stVehSpdECFlg)  "stVehSpdECFlg"

== system LKAS_AutoSave_DF_20220414_1924_SW62/LKAS/LL/LLOn/LL State Determination (LLStateDet)/LL State Machine Conditions (LLSMCon)/Fault Condition (FaultC)/16Bits_Set2 ==
  Bit0 : Inport  OutDataTypeStr=boolean
  Bit1 : Inport  Port=2  OutDataTypeStr=boolean
  Bit2 : Inport  Port=3  OutDataTypeStr=boolean
  Bit3 : Inport  Port=4  OutDataTypeStr=boolean
  Bit4 : Inport  Port=5  OutDataTypeStr=boolean
  Bit5 : Inport  Port=6  OutDataTypeStr=boolean
  Bit6 : Inport  Port=7  OutDataTypeStr=boolean
  Bit7 : Inport  Port=8  OutDataTypeStr=boolean
  Bit8 : Inport  Port=9  OutDataTypeStr=boolean
  Bit9 : Inport  Port=10  OutDataTypeStr=boolean
  Bit10 : Inport  Port=11  OutDataTypeStr=boolean
  Bit11 : Inport  Port=12  OutDataTypeStr=boolean
  Bit12 : Inport  Port=13  OutDataTypeStr=boolean
  Bit13 : Inport  Port=14  OutDataTypeStr=boolean
  Bit14 : Inport  Port=15  OutDataTypeStr=boolean
  Bit15 : Inport  Port=16  OutDataTypeStr=boolean
  Bit16 : Inport  Port=17  OutDataTypeStr=boolean
  Bit17 : Inport  Port=18  OutDataTypeStr=boolean
  Bit18 : Inport  Port=19  OutDataTypeStr=boolean
  Bit19 : Inport  Port=20  OutDataTypeStr=boolean
  Bit20 : Inport  Port=21  OutDataTypeStr=boolean
  Bit21 : Inport  Port=22  OutDataTypeStr=boolean
  Bit22 : Inport  Port=23  OutDataTypeStr=boolean
  Bit23 : Inport  Port=24  OutDataTypeStr=boolean
  8Bits_Set : Subsystem
  8Bits_Set1 : Subsystem
  8Bits_Set2 : Subsystem
  Add : Sum  Inputs=+++  AccumDataTypeStr=uint32
  Data Type Conversion : DataTypeConversion  OutDataTypeStr=uint32
  Data Type Conversion1 : DataTypeConversion  OutDataTypeStr=uint32
  Data Type Conversion2 : DataTypeConversion  OutDataTypeStr=uint32
  Shift Arithmetic : ArithShift  BitShiftNumber=8  BitShiftDirection=Left
  Shift Arithmetic1 : ArithShift  BitShiftNumber=16  BitShiftDirection=Left
  Index_32Bits : Outport  OutDataTypeStr=uint32
  wires:
  Shift Arithmetic1/1 -> Add/3
  Data Type Conversion2/1 -> Shift Arithmetic1/1
  Bit21/1 -> 8Bits_Set2/6(Bit5)
  Bit16/1 -> 8Bits_Set2/1(Bit0)
  Bit17/1 -> 8Bits_Set2/2(Bit1)
  Bit23/1 -> 8Bits_Set2/8(Bit7)
  8Bits_Set2/1(Index_8Bits) -> Data Type Conversion2/1
  Bit20/1 -> 8Bits_Set2/5(Bit4)
  Bit19/1 -> 8Bits_Set2/4(Bit3)
  Bit18/1 -> 8Bits_Set2/3(Bit2)
  Bit22/1 -> 8Bits_Set2/7(Bit6)
  Bit15/1 -> 8Bits_Set1/8(Bit7)
  Bit14/1 -> 8Bits_Set1/7(Bit6)
  Bit13/1 -> 8Bits_Set1/6(Bit5)
  Bit12/1 -> 8Bits_Set1/5(Bit4)
  Bit11/1 -> 8Bits_Set1/4(Bit3)
  Bit10/1 -> 8Bits_Set1/3(Bit2)
  Bit9/1 -> 8Bits_Set1/2(Bit1)
  Bit8/1 -> 8Bits_Set1/1(Bit0)
  Bit7/1 -> 8Bits_Set/8(Bit7)
  Bit6/1 -> 8Bits_Set/7(Bit6)
  Bit5/1 -> 8Bits_Set/6(Bit5)
  Bit4/1 -> 8Bits_Set/5(Bit4)
  Bit3/1 -> 8Bits_Set/4(Bit3)
  Bit2/1 -> 8Bits_Set/3(Bit2)
  Bit1/1 -> 8Bits_Set/2(Bit1)
  Bit0/1 -> 8Bits_Set/1(Bit0)
  Data Type Conversion1/1 -> Shift Arithmetic/1
  Data Type Conversion/1 -> Add/1
  Add/1 -> Index_32Bits/1
  8Bits_Set/1(Index_8Bits) -> Data Type Conversion/1
  Shift Arithmetic/1 -> Add/2
  8Bits_Set1/1(Index_8Bits) -> Data Type Conversion1/1

== system LKAS_AutoSave_DF_20220414_1924_SW62/LKAS/LL/LLOn/LL State Determination (LLStateDet)/LL State Machine Conditions (LLSMCon)/Fault Condition (FaultC)/Count_5s1 ==
  SampleTime : Inport
  Add : Sum
  Constant1 : Constant  Value=5  OutDataTypeStr=uint16
  Memory : Memory  InheritSampleTime=on
  Relational Operator : RelationalOperator  OutDataTypeStr=boolean  RndMeth=Simplest
  Saturation : Saturate  UpperLimit=11  LowerLimit=0
      settings: AttributesFormatString="Min = %<LowerLimit>  Max = %<UpperLimit>"
  Out : Outport  OutputWhenDisabled=reset  InitialOutput=0
      settings: AttributesFormatString=%<OutputWhenDisabled> = %<InitialOutput>
  wires:
  Constant1/1 -> Relational Operator/2
  Relational Operator/1 -> Out/1
  Saturation/1 -> Memory/1, Relational Operator/1
  SampleTime/1 -> Add/2
  Add/1 -> Saturation/1
  Memory/1 -> Add/1

== system LKAS_AutoSave_DF_20220414_1924_SW62/LKAS/LL/LL Inputs Mapping/bsLaneInfo/LanesReconstruct /RoadSide Offset/Road Width Calculation (RoadWCal)/Average Filter (AvrgFlt)1 ==
  In : Inport
  PtsNum : Inport  Port=2
  Add1 : Sum
  Add2 : Sum  Inputs=-+
  Constant : Constant  OutDataTypeStr=single
  Constant1 : Constant  OutDataTypeStr=single
  Divide : Product  Inputs=**
  Divide1 : Product  Inputs=**
  Divide2 : Product  Inputs=*/
  Memory : Memory  InitialCondition=3.2  InheritSampleTime=on
  Saturation : Saturate  UpperLimit=10000  LowerLimit=1  OutDataTypeStr=single
      settings: AttributesFormatString="Min = %<LowerLimit>  Max = %<UpperLimit>"
  Out : Outport
  wires:
  Constant1/1 -> Divide2/1
  Saturation/1 -> Divide2/2
  Memory/1 -> Divide1/2
  Divide2/1 -> Divide/2, Add2/1
  Add1/1 -> Memory/1, Out/1
  Divide1/1 -> Add1/2
  Add2/1 -> Divide1/1
  Constant/1 -> Add2/2
  Divide/1 -> Add1/1
  PtsNum/1 -> Saturation/1
  In/1 -> Divide/1

== system LKAS_AutoSave_DF_20220414_1924_SW62/LKAS/LL/LLOn/LKA/LKA Motion Planning (LKAMP) /Motion Planning Input Processing (MPInP)/Lane Information Selection (LaneInfoSel)/If Action Subsystem1 ==
  In1 : Inport
  Action Port : ActionPort  InitializeStates=reset  ActionType=elseif
      settings: AttributesFormatString=states = %<InitializeStates>
  Out1 : Outport
      settings: AttributesFormatString=%<OutputWhenDisabled> = %<InitialOutput>
  wires:
  In1/1 -> Out1/1

== system LKAS_AutoSave_DF_20220414_1924_SW62/LKAS/LL/LLOn/LKA/LKA Motion Planning (LKAMP) /Motion Planning Input Processing (MPInP)/Lane Information Selection (LaneInfoSel)/If Action Subsystem2 ==
  In1 : Inport
  Action Port : ActionPort  InitializeStates=reset  ActionType=then
      settings: AttributesFormatString=states = %<InitializeStates>
  Out1 : Outport
      settings: AttributesFormatString=%<OutputWhenDisabled> = %<InitialOutput>
  wires:
  In1/1 -> Out1/1

== system LKAS_AutoSave_DF_20220414_1924_SW62/LKAS/LL/LLOn/LKA/LKA Motion Planning (LKAMP) /Motion Planning Input Processing (MPInP)/Lane Information Selection (LaneInfoSel)/If Action Subsystem3 ==
  Action Port : ActionPort  InitializeStates=reset  ActionType=else
      settings: AttributesFormatString=states = %<InitializeStates>
  Constant : Constant  Value=0  OutDataTypeStr=single
  Out1 : Outport
      settings: AttributesFormatString=%<OutputWhenDisabled> = %<InitialOutput>
  wires:
  Constant/1 -> Out1/1

== system LKAS_AutoSave_DF_20220414_1924_SW62/LKAS/LL/LLOn/LKA/LKA Motion Planning (LKAMP) /Motion Planning Input Processing (MPInP)/Lane Information Selection (LaneInfoSel)1/If Action Subsystem1 ==
  In1 : Inport
  Action Port : ActionPort  InitializeStates=reset  ActionType=elseif
      settings: AttributesFormatString=states = %<InitializeStates>
  Out1 : Outport
      settings: AttributesFormatString=%<OutputWhenDisabled> = %<InitialOutput>
  wires:
  In1/1 -> Out1/1

== system LKAS_AutoSave_DF_20220414_1924_SW62/LKAS/LL/LLOn/LKA/LKA Motion Planning (LKAMP) /Motion Planning Input Processing (MPInP)/Lane Information Selection (LaneInfoSel)1/If Action Subsystem2 ==
  In1 : Inport
  Action Port : ActionPort  InitializeStates=reset  ActionType=then
      settings: AttributesFormatString=states = %<InitializeStates>
  Out1 : Outport
      settings: AttributesFormatString=%<OutputWhenDisabled> = %<InitialOutput>
  wires:
  In1/1 -> Out1/1

== system LKAS_AutoSave_DF_20220414_1924_SW62/LKAS/LL/LLOn/LKA/LKA Motion Planning (LKAMP) /Motion Planning Input Processing (MPInP)/Lane Information Selection (LaneInfoSel)1/If Action Subsystem3 ==
  Action Port : ActionPort  InitializeStates=reset  ActionType=else
      settings: AttributesFormatString=states = %<InitializeStates>
  Constant : Constant  Value=0  OutDataTypeStr=single
  Out1 : Outport
      settings: AttributesFormatString=%<OutputWhenDisabled> = %<InitialOutput>
  wires:
  Constant/1 -> Out1/1

== system LKAS_AutoSave_DF_20220414_1924_SW62/LKAS/LL/LLOn/LKA/LKA Motion Planning (LKAMP) /Motion Planning Input Processing (MPInP)/Lane Information Selection (LaneInfoSel)2/If Action Subsystem1 ==
  In1 : Inport
  Action Port : ActionPort  InitializeStates=reset  ActionType=elseif
      settings: AttributesFormatString=states = %<InitializeStates>
  Out1 : Outport
      settings: AttributesFormatString=%<OutputWhenDisabled> = %<InitialOutput>
  wires:
  In1/1 -> Out1/1

== system LKAS_AutoSave_DF_20220414_1924_SW62/LKAS/LL/LLOn/LKA/LKA Motion Planning (LKAMP) /Motion Planning Input Processing (MPInP)/Lane Information Selection (LaneInfoSel)2/If Action Subsystem2 ==
  In1 : Inport
  Action Port : ActionPort  InitializeStates=reset  ActionType=then
      settings: AttributesFormatString=states = %<InitializeStates>
  Out1 : Outport
      settings: AttributesFormatString=%<OutputWhenDisabled> = %<InitialOutput>
  wires:
  In1/1 -> Out1/1

== system LKAS_AutoSave_DF_20220414_1924_SW62/LKAS/LL/LLOn/LKA/LKA Motion Planning (LKAMP) /Motion Planning Input Processing (MPInP)/Lane Information Selection (LaneInfoSel)2/If Action Subsystem3 ==
  Action Port : ActionPort  InitializeStates=reset  ActionType=else
      settings: AttributesFormatString=states = %<InitializeStates>
  Constant : Constant  Value=0  OutDataTypeStr=single
  Out1 : Outport
      settings: AttributesFormatString=%<OutputWhenDisabled> = %<InitialOutput>
  wires:
  Constant/1 -> Out1/1

== system LKAS_AutoSave_DF_20220414_1924_SW62/LKAS/LL/LLOn/LKA/LKA Motion Planning (LKAMP) /Motion Planning Input Processing (MPInP)/Lane Information Selection (LaneInfoSel)3/If Action Subsystem1 ==
  In1 : Inport
  Action Port : ActionPort  InitializeStates=reset  ActionType=elseif
      settings: AttributesFormatString=states = %<InitializeStates>
  Out1 : Outport
      settings: AttributesFormatString=%<OutputWhenDisabled> = %<InitialOutput>
  wires:
  In1/1 -> Out1/1

== system LKAS_AutoSave_DF_20220414_1924_SW62/LKAS/LL/LLOn/LKA/LKA Motion Planning (LKAMP) /Motion Planning Input Processing (MPInP)/Lane Information Selection (LaneInfoSel)3/If Action Subsystem2 ==
  In1 : Inport
  Action Port : ActionPort  InitializeStates=reset  ActionType=then
      settings: AttributesFormatString=states = %<InitializeStates>
  Out1 : Outport
      settings: AttributesFormatString=%<OutputWhenDisabled> = %<InitialOutput>
  wires:
  In1/1 -> Out1/1

== system LKAS_AutoSave_DF_20220414_1924_SW62/LKAS/LL/LLOn/LKA/LKA Motion Planning (LKAMP) /Motion Planning Input Processing (MPInP)/Lane Information Selection (LaneInfoSel)3/If Action Subsystem3 ==
  Action Port : ActionPort  InitializeStates=reset  ActionType=else
      settings: AttributesFormatString=states = %<InitializeStates>
  Constant : Constant  Value=0  OutDataTypeStr=single
  Out1 : Outport
      settings: AttributesFormatString=%<OutputWhenDisabled> = %<InitialOutput>
  wires:
  Constant/1 -> Out1/1

== system LKAS_AutoSave_DF_20220414_1924_SW62/LKAS/LL/LLOn/LKA/LKA Motion Planning (LKAMP) /Motion Planning Input Processing (MPInP)/Lane Information Selection (LaneInfoSel)4/If Action Subsystem1 ==
  In1 : Inport
  Action Port : ActionPort  InitializeStates=reset  ActionType=elseif
      settings: AttributesFormatString=states = %<InitializeStates>
  Out1 : Outport
      settings: AttributesFormatString=%<OutputWhenDisabled> = %<InitialOutput>
  wires:
  In1/1 -> Out1/1

== system LKAS_AutoSave_DF_20220414_1924_SW62/LKAS/LL/LLOn/LKA/LKA Motion Planning (LKAMP) /Motion Planning Input Processing (MPInP)/Lane Information Selection (LaneInfoSel)4/If Action Subsystem2 ==
  In1 : Inport
  Action Port : ActionPort  InitializeStates=reset  ActionType=then
      settings: AttributesFormatString=states = %<InitializeStates>
  Out1 : Outport
      settings: AttributesFormatString=%<OutputWhenDisabled> = %<InitialOutput>
  wires:
  In1/1 -> Out1/1

== system LKAS_AutoSave_DF_20220414_1924_SW62/LKAS/LL/LLOn/LKA/LKA Motion Planning (LKAMP) /Motion Planning Input Processing (MPInP)/Lane Information Selection (LaneInfoSel)4/If Action Subsystem3 ==
  Action Port : ActionPort  InitializeStates=reset  ActionType=else
      settings: AttributesFormatString=states = %<InitializeStates>
  Constant : Constant  Value=0  OutDataTypeStr=single
  Out1 : Outport
      settings: AttributesFormatString=%<OutputWhenDisabled> = %<InitialOutput>
  wires:
  Constant/1 -> Out1/1

== system LKAS_AutoSave_DF_20220414_1924_SW62/LKAS/LL/LLOn/LKA/LKA Motion Planning (LKAMP) /Motion Planning Input Processing (MPInP)/Signal Latching/if action  ==
  In : Inport
  Action Port : ActionPort  InitializeStates=reset  ActionType=then
  Out : Outport
  wires:
  In/1 -> Out/1

== system LKAS_AutoSave_DF_20220414_1924_SW62/LKAS/LL/LLOn/LKA/LKA Motion Planning (LKAMP) /Motion Planning Input Processing (MPInP)/Signal Latching2/if action  ==
  In : Inport
  Action Port : ActionPort  InitializeStates=reset  ActionType=then
  Out : Outport
  wires:
  In/1 -> Out/1

== system LKAS_AutoSave_DF_20220414_1924_SW62/LKAS/LL/LLOn/LKA/LKA Motion Planning (LKAMP) /Motion Planning Input Processing (MPInP)/Signal Latching3/if action  ==
  In : Inport
  Action Port : ActionPort  InitializeStates=reset  ActionType=then
  Out : Outport
  wires:
  In/1 -> Out/1

== system LKAS_AutoSave_DF_20220414_1924_SW62/LKAS/LL/LLOn/LKA/LKA Motion Planning (LKAMP) /Motion Planning Input Processing (MPInP)/Signal Latching4/if action  ==
  In : Inport
  Action Port : ActionPort  InitializeStates=reset  ActionType=then
  Out : Outport
  wires:
  In/1 -> Out/1

== system LKAS_AutoSave_DF_20220414_1924_SW62/LKAS/LL/LLOn/LKA/LKA Motion Planning (LKAMP) /Motion Planning Input Processing (MPInP)/Signal Latching5/if action  ==
  In : Inport
  Action Port : ActionPort  InitializeStates=reset  ActionType=then
  Out : Outport
  wires:
  In/1 -> Out/1

== system LKAS_AutoSave_DF_20220414_1924_SW62/LKAS/LL/LLOn/LKA/LKA Motion Planning (LKAMP) /Motion Planning Input Processing (MPInP)/Signal Latching6/if action  ==
  In : Inport
  Action Port : ActionPort  InitializeStates=reset  ActionType=then
  Out : Outport
  wires:
  In/1 -> Out/1

== system LKAS_AutoSave_DF_20220414_1924_SW62/LKAS/LL/LLOn/LKA/LKA Motion Planning (LKAMP) /Motion Planning Input Processing (MPInP)/Signal Latching7/if action  ==
  In : Inport
  Action Port : ActionPort  InitializeStates=reset  ActionType=then
  Out : Outport
  wires:
  In/1 -> Out/1

== system LKAS_AutoSave_DF_20220414_1924_SW62/LKAS/LL/LLOn/LKA/LKA Motion Planning (LKAMP) /Motion Planning Input Processing (MPInP)/Subsystem/If Action Subsystem1 ==
  Action Port : ActionPort  InitializeStates=reset  ActionType=elseif
      settings: AttributesFormatString=states = %<InitializeStates>
  Constant : Constant  OutDataTypeStr=single
  Out1 : Outport
      settings: AttributesFormatString=%<OutputWhenDisabled> = %<InitialOutput>
  wires:
  Constant/1 -> Out1/1
